simulink model "GERBOX"  (R2023a)
settings: Solver=VariableStepAuto  StartTime=0.0  StopTime=1  RelTol=1e-3
settings Model: Creator=ycheb  LastModifiedBy=ycheb

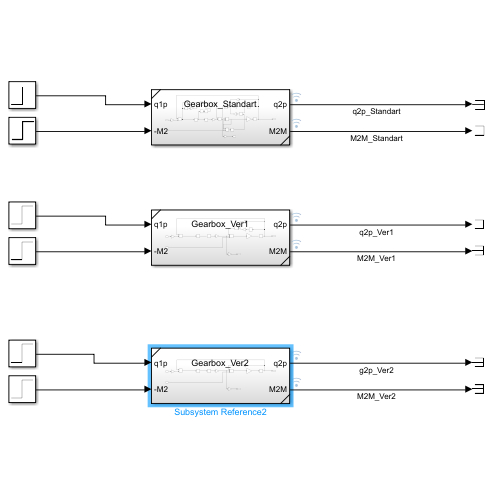
[thumbnail: Simulink's stored preview of the top-level diagram]
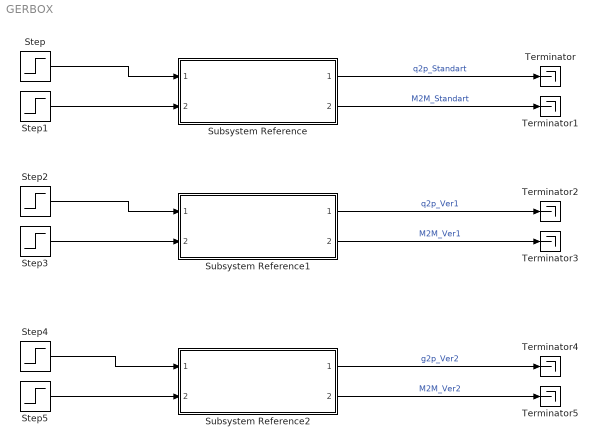
== system GERBOX ==
  Step{,1..5} (6 alike) : Step  Time=0  SampleTime=0
  Subsystem Reference : Subsystem  ReferencedSubsystem=Gearbox_Standart
  Subsystem Reference1 : Subsystem  ReferencedSubsystem=Gearbox_Ver1
  Subsystem Reference2 : Subsystem  ReferencedSubsystem=Gearbox_Ver2
  Terminator{,1..5} (6 alike) : Terminator
  wires:
  Step1/1 -> Subsystem Reference/2
  Step/1 -> Subsystem Reference/1
  Subsystem Reference/2 -> Terminator1/1  "M2M_Standart"
  Subsystem Reference/1 -> Terminator/1  "q2p_Standart"
  Subsystem Reference1/2 -> Terminator3/1  "M2M_Ver1"
  Step2/1 -> Subsystem Reference1/1
  Step3/1 -> Subsystem Reference1/2
  Subsystem Reference1/1 -> Terminator2/1  "q2p_Ver1"
  Subsystem Reference2/1 -> Terminator4/1  "g2p_Ver2"
  Subsystem Reference2/2 -> Terminator5/1  "M2M_Ver2"
  Step4/1 -> Subsystem Reference2/1
  Step5/1 -> Subsystem Reference2/2
